simulink model "butterfly_matlab_to_c"  (R2020a)
settings: Solver=FixedStepAuto  StartTime=0.0  StopTime=30  FixedStep=1/120/10  MaxStep=0.01  RelTol=1e-3
undefined symbols (not defined in the file or in its folder): bf
settings Model: SimulationMode=accelerator  Creator=g-oft  LastModifiedBy=g-oft
settings DataIOCC: SaveFormat=StructureWithTime
settings OptimizationCC: OptimizeBlockIOStorage=off  OptimizeDataStoreBuffers=off  BusAssignmentInplaceUpdate=off
settings DebuggingCC: SFUnexpectedBacktrackingDiag=warning  SFNoUnconditionalDefaultTransitionDiag=warning
settings RTWCC: GenerateReport=on  BuildConfiguration=Debug  LaunchReport=on
settings CodeAppCC: ForceParamTrailComments=on  MATLABSourceComments=on  EnableCustomComments=on
settings GRTTargetCC: CombineSignalStateStructs=on  SupportVariableSizeSignals=on  RTWCAPISignals=on  RTWCAPIParams=on  RTWCAPIStates=on  MultiInstanceErrorCode=Warning

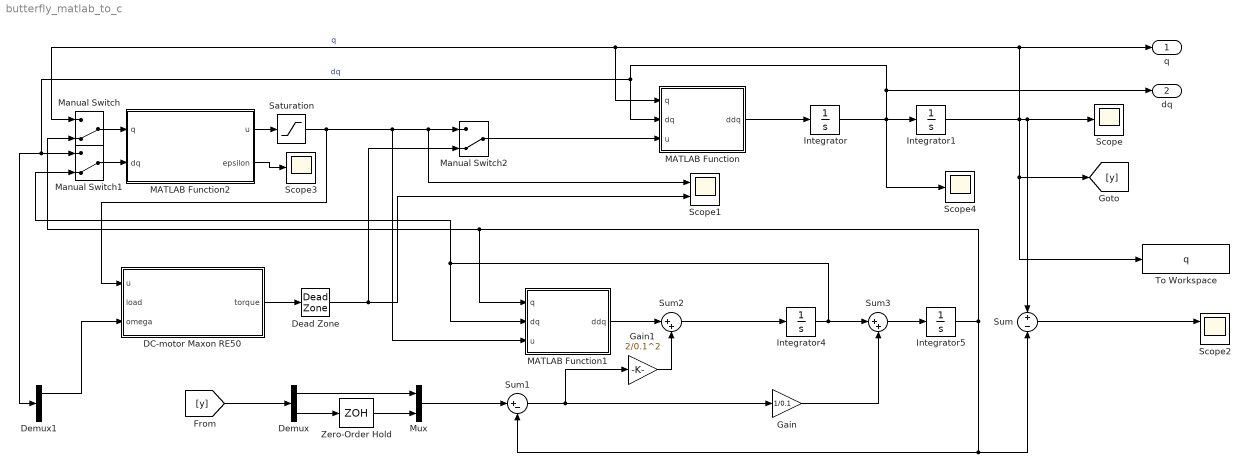
== system butterfly_matlab_to_c ==
  DC-motor Maxon RE50 : Subsystem
  Dead Zone : DeadZone  LowerValue=-5e-3  UpperValue=5e-3  SaturateOnIntegerOverflow=on
  Demux : Demux  Outputs=2
  Demux1 : Demux  Outputs=2
  Gain : Gain  Gain=1/0.1
  Gain1 : Gain  Gain=2/0.1^2
  Integrator : Integrator  InitialCondition=[bf.get_dtheta(0)*bf.function_for_dphi(0);bf.function_for_dphi(0)]
  Integrator1 : Integrator  InitialCondition=[0;0]
  Integrator4 : Integrator  InitialCondition=[0.3;0]
  Integrator5 : Integrator  InitialCondition=[0.1;0]
  MATLAB Function : MATLAB Function  TreatAsAtomicUnit=on
  MATLAB Function1 : MATLAB Function  TreatAsAtomicUnit=on
  MATLAB Function2 : MATLAB Function  TreatAsAtomicUnit=on
  Manual Switch : ManualSwitch  CurrentSetting=0
  Manual Switch1 : ManualSwitch  CurrentSetting=0
  Manual Switch2 : ManualSwitch  CurrentSetting=0
  Mux : Mux  Inputs=2
  Saturation : Saturate  UpperLimit=10  LowerLimit=-10
  Scope : Scope
  Scope1 : Scope  NumInputPorts=2
  Scope2 : Scope  NumInputPorts=2
  Scope3 : Scope
  Scope4 : Scope
  Sum : Sum  Inputs=+-
  Sum1 : Sum  Inputs=|+-
  Sum2 : Sum  Inputs=|++
  Sum3 : Sum  Inputs=|++
  To Workspace : ToWorkspace  VariableName=q  SampleTime=-1
  Zero-Order Hold : ZeroOrderHold  SampleTime=1/120
  q : Outport  SignalName=q
  dq : Outport  Port=2  SignalName=dq
  wires:
  Integrator/1 -> Scope4/1, Integrator1/1, dq/1, Demux1/1, Manual Switch1/1, MATLAB Function/2(dq)  "dq"
  MATLAB Function/1(ddq) -> Integrator/1
  Integrator1/1 -> Sum/1, Scope/1, [y], To Workspace/1, q/1, Manual Switch/1, MATLAB Function/1(q)  "q"
  Integrator4/1 -> MATLAB Function1/2(dq), Manual Switch1/2, Sum3/1
  Sum3/1 -> Integrator5/1
  Integrator5/1 -> Sum/2, Sum1/2, MATLAB Function1/1(q), Manual Switch/2
  Gain1/1 -> Sum2/2
  Gain/1 -> Sum3/2
  MATLAB Function1/1(ddq) -> Sum2/1
  Sum1/1 -> Gain1/1, Gain/1
  Manual Switch1/1 -> MATLAB Function2/2(dq)
  Manual Switch/1 -> MATLAB Function2/1(q)
  Sum2/1 -> Integrator4/1
  Sum/1 -> Scope2/1
  MATLAB Function2/1(u) -> Saturation/1
  DC-motor Maxon RE50/1(torque) -> Dead Zone/1
  Manual Switch2/1 -> MATLAB Function/3(u)
  Saturation/1 -> DC-motor Maxon RE50/1(u), MATLAB Function1/3(u), Scope1/1, Manual Switch2/1
  Demux1/1 -> DC-motor Maxon RE50/3(omega)
  Mux/1 -> Sum1/1
  [y] -> Demux/1
  Zero-Order Hold/1 -> Mux/2
  Demux/2 -> Zero-Order Hold/1
  Demux/1 -> Mux/1
  MATLAB Function2/2(epsilon) -> Scope3/1
  Dead Zone/1 -> Manual Switch2/2, Scope1/2

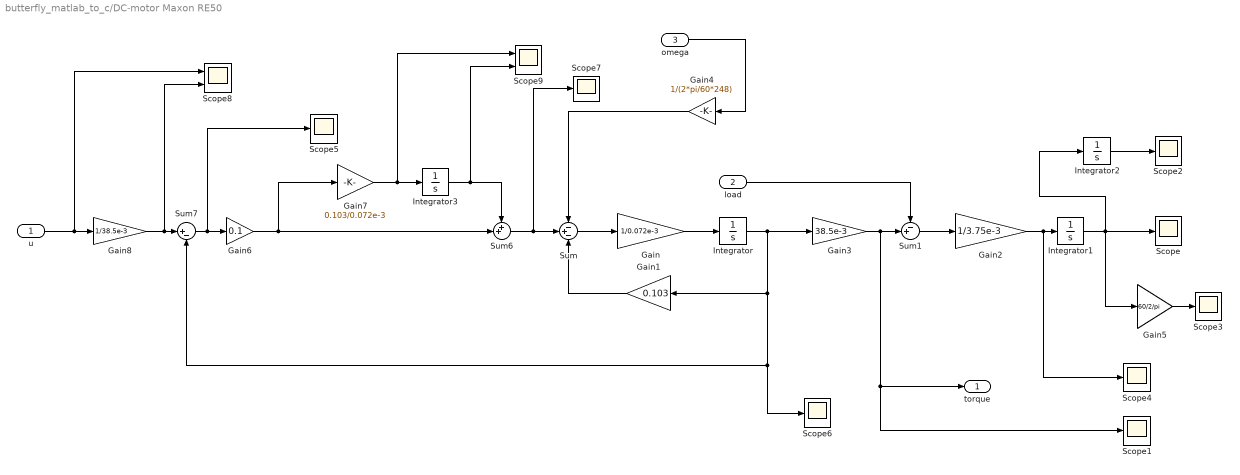
== system butterfly_matlab_to_c/DC-motor Maxon RE50 ==
  u : Inport
  load : Inport  Port=2
  omega : Inport  Port=3
  Gain : Gain  Gain=1/0.072e-3
  Gain1 : Gain  Gain=0.103
  Gain2 : Gain  Gain=1/3.75e-3
  Gain3 : Gain  Gain=38.5e-3
  Gain4 : Gain  Gain=1/(2*pi/60*248)
  Gain5 : Gain  Gain=60/2/pi
  Gain6 : Gain  Gain=0.1
  Gain7 : Gain  Gain=0.103/0.072e-3
  Gain8 : Gain  Gain=1/38.5e-3
  Integrator{,1..3} (4 alike) : Integrator
  Scope{,1..7} (8 alike) : Scope
  Scope8 : Scope  NumInputPorts=2
  Scope9 : Scope  NumInputPorts=2
  Sum : Sum  Inputs=-+-
  Sum1 : Sum  Inputs=-+|
  Sum6 : Sum  Inputs=++|
  Sum7 : Sum  Inputs=|+-
  torque : Outport
  wires:
  Sum/1 -> Gain/1
  Gain/1 -> Integrator/1
  Gain1/1 -> Sum/3
  Sum1/1 -> Gain2/1
  Gain2/1 -> Scope4/1, Integrator1/1
  Gain3/1 -> torque/1, Scope1/1, Sum1/2
  Integrator1/1 -> Gain5/1, Scope/1, Integrator2/1
  Gain4/1 -> Sum/1
  Integrator2/1 -> Scope2/1
  Gain5/1 -> Scope3/1
  Integrator/1 -> Gain1/1, Scope6/1, Sum7/2, Gain3/1
  Integrator3/1 -> Scope9/2, Sum6/1
  Gain6/1 -> Gain7/1, Sum6/2
  Sum7/1 -> Scope5/1, Gain6/1
  Sum6/1 -> Scope7/1, Sum/2
  u/1 -> Scope8/1, Gain8/1
  Gain8/1 -> Scope8/2, Sum7/1
  load/1 -> Sum1/1
  Gain7/1 -> Scope9/1, Integrator3/1
  omega/1 -> Gain4/1

== matlab function butterfly_matlab_to_c/MATLAB Function ==
  settings: updateMethod=DISCRETE
  data: q input; dq input; u input; ddq output
function ddq = calculate_ddq(q,dq,u)
    persistent solutions
    if isempty(solutions)
        solutions = coder.load('solutions_riccati_and_dphi');
    end
    n_varphi = 5000;
    a = 0.1095; %Constant for describing the butterfly frame
    b = 0.0405; %Constant for describing the butterfly frame
    g = 9.81; %Gravity
    J_s = 5.48e-7; %Mass moment of inertia of the ball
    J_f = 1.581e-2; %Mass moment of inertia of the frame, from article.
    m_b = 3.0e-3; %Mass of the ball
    R_b = sqrt(16.55e-3^2-12.5e-3^2); %Radius of the ball
    
    %% Functions relating phi and varphi:
   
    % Temporary using phi = varphi;
    varphi = q(2);
    vartheta = q(1);
    phi = solutions.varphi_to_phi(1,floor(mod(varphi,2*pi)*n_varphi/2/pi)+1);
    

    %% e_phi 
    e_phi = [sin(phi);cos(phi);0];
    d_e_phi = [cos(phi);-sin(phi);0];
    dd_e_phi = [-sin(phi);-cos(phi);0];
    ddd_e_phi = [-cos(phi);sin(phi);0];
    
    %% Delta
    delta = (a-b*cos(2*phi));
    delta_v = delta*e_phi;
    d_delta = b*2*sin(2*phi);
    dd_delta = b*4*cos(2*phi);
    ddd_delta = -b*8*sin(2*phi);
    d_delta_v = d_delta*e_phi+delta*d_e_phi;
    dd_delta_v = dd_delta*e_phi+2*d_delta*d_e_phi+delta*dd_e_phi;
    ddd_delta_v = ddd_delta*e_phi+ 3*dd_delta*d_e_phi + ...
        3*d_delta*dd_e_phi + delta*ddd_e_phi;
    norm_d_delta_v = sqrt(d_delta^2+delta^2);
    
    %% Tau
    tau = d_delta_v/norm_d_delta_v;
    d_tau = dd_delta_v/norm_d_delta_v - d_delta_v*d_delta_v'*dd_delta_v/norm_d_delta_v^3;
    dd_tau = ddd_delta_v/norm_d_delta_v - dd_delta_v*d_delta_v'*dd_delta_v/norm_d_delta_v^3 - ...
        (dd_delta_v*d_delta_v'*dd_delta_v+d_delta_v*(dd_delta_v'*dd_delta_v)+d_delta_v*d_delta_v'*ddd_delta_v)/...
        norm_d_delta_v^3 + d_delta_v*d_delta_v'*dd_delta_v*3*d_delta_v'*dd_delta_v/norm_d_delta_v^5;
    %% Normal vector:
    normal = [0 -1 0;1 0 0;0 0 0]*tau;
    d_normal = [0 -1 0;1 0 0;0 0 0]*d_tau;
    dd_normal = [0 -1 0;1 0 0;0 0 0]*dd_tau;
    

    %% Rho :
    rho = delta_v + R_b*normal;
    d_rho = d_delta_v + R_b*d_normal;
    dd_rho = dd_delta_v + R_b*dd_normal;
    
    %% Need to find varphi = g(phi)
    gamma = delta_v'*[1;0;0]-R_b*tau'*[0;1;0];
    psi = delta_v'*[0;1;0]+R_b*tau'*[1;0;0];
    d_gamma = d_delta_v'*[1;0;0]-R_b*d_tau'*[0;1;0];
    d_psi = d_delta_v'*[0;1;0]+R_b*d_tau'*[1;0;0];
    dd_gamma = dd_delta_v'*[1;0;0]-R_b*dd_tau'*[0;1;0];
    dd_psi = dd_delta_v'*[0;1;0]+R_b*dd_tau'*[1;0;0];
    %func_g = atan2(gamma, psi);
    d_func_g = (d_gamma*psi-d_psi*gamma)/(gamma^2+psi^2);
    dd_func_g = (dd_gamma*psi-dd_psi*gamma)/(psi^2+gamma^2)-(d_gamma*psi-d_psi*gamma)*(2*gamma*d_gamma+2*psi*d_psi)/(gamma^2+psi^2)^2;
    
    %% s
    d_s = norm(d_rho)/d_func_g;
    dd_s = d_rho'*dd_rho/norm(d_rho)/d_func_g^2 - norm(d_rho)*dd_func_g/d_func_g^3;
    
    %% s_f:
    d_sf = norm_d_delta_v/d_func_g;
    dd_sf = d_delta_v'*dd_delta_v/norm_d_delta_v/d_func_g - norm_d_delta_v*dd_func_g/d_func_g^3;
    
    %% Kappa:
    kappa = dd_rho/d_func_g^2/d_s^2;
    
    %% Rotations:
    R = [cos(vartheta) -sin(vartheta) 0;sin(vartheta) cos(vartheta) 0;0 0 1];
    dR = [-sin(vartheta) -cos(vartheta) 0;cos(vartheta) -sin(vartheta) 0;0 0 0];
    
    rhoxtau = cross(rho,tau);
    rhoxkappa = cross(rho,kappa);
    
    m_11 = m_b*(rho'*rho+J_s/m_b+J_f/m_b);
    m_12 = m_b*(d_s*rhoxtau(3)-d_sf*J_s/R_b/m_b);
    m_22 = m_b*(d_s^2+d_sf^2*J_s/R_b^2/m_b);
    M = [m_11 m_12;m_12 m_22];
    
    c_11 = m_b*rho'*tau*d_s*dq(2);
    c_12 = m_b*(rho'*tau*d_s*dq(1)+(dd_s*rhoxtau(3)-dd_sf*J_s/R_b/m_b+d_s^2*rhoxkappa(3))*dq(2));
    c_21 = -m_b*rho'*tau*d_s*dq(1);
    c_22 = m_b*(d_s*dd_s+d_sf*dd_sf*J_s/R_b^2/m_b)*dq(2);
    C = [c_11 c_12;c_21 c_22];
    
    
    G = m_b*[[0 g 0]*dR*rho;[0 g 0]*R*tau*d_s];

    
ddq = M\(-C*[dq(1);dq(2)]-G+[u;0]);

== matlab function butterfly_matlab_to_c/MATLAB Function2 ==
  settings: updateMethod=DISCRETE
  data: q input; u output; dq input; epsilon output
function [u,epsilon] = controller(q,dq)
    
    persistent solutions
    if isempty(solutions)
        solutions = coder.load('solutions_riccati_and_dphi');
    end
    n_varphi = 5000;
    n_riccati_sol = 5000;
    a = 0.1095; %Constant for describing the butterfly frame
    b = 0.0405; %Constant for describing the butterfly frame
    g = 9.81; %Gravity
    J_s = 5.48e-7; %Mass moment of inertia of the ball
    J_f = 1.581e-2; %Mass moment of inertia of the frame, from article.
    m_b = 3.0e-3; %Mass of the ball
    R_b = sqrt(16.55e-3^2-12.5e-3^2); %Radius of the ball
    

    varphi = q(2);

    c1= -6.023940e+01; c2= 9.115470e-03; c3= 1.941337e-03; c4= 1.731620e-03; c5= 7.253528e-04;
    Theta = c1*atan(c2*sin(2*varphi)+c3*sin(4*varphi)+c4*sin(6*varphi)+c5*sin(8*varphi))+varphi;
    d_Theta = c1*(2*c2*cos(2*varphi) + 4*c3*cos(4*varphi) + 6*c4*cos(6*varphi) + 8*c5*cos(8*varphi))/((c2*sin(2*varphi) + c3*sin(4*varphi) + c4*sin(6*varphi) + c5*sin(8*varphi))^2 + 1) + 1;
    dd_Theta = c1*(-4*c2*sin(2*varphi) - 16*c3*sin(4*varphi) - 36*c4*sin(6*varphi) - 64*c5*sin(8*varphi))/((c2*sin(2*varphi) + c3*sin(4*varphi) + c4*sin(6*varphi) + c5*sin(8*varphi))^2 + 1) - 2*c1*(2*c2*cos(2*varphi) + 4*c3*cos(4*varphi) + 6*c4*cos(6*varphi) + 8*c5*cos(8*varphi))^2*(c2*sin(2*varphi) + c3*sin(4*varphi) + c4*sin(6*varphi) + c5*sin(8*varphi))/((c2*sin(2*varphi) + c3*sin(4*varphi) + c4*sin(6*varphi) + c5*sin(8*varphi))^2 + 1)^2;
    
%     c = [0.0024   -0.0383    0.2090   -0.4568    1.3214    0.0055];
%     x = varphi;
%     phi = varphi;%c*[x^5;x^4;x^3;x^2;x;1];
    phi = solutions.varphi_to_phi(1,floor(mod(varphi,2*pi)*n_varphi/2/pi)+1);
    vartheta = Theta;
    d_vartheta = d_Theta*dq(2);
    
    %% e_phi 
    e_phi = [sin(phi);cos(phi);0];
    d_e_phi = [cos(phi);-sin(phi);0];
    dd_e_phi = [-sin(phi);-cos(phi);0];
    ddd_e_phi = [-cos(phi);sin(phi);0];
    
    %% Delta
    delta = (a-b*cos(2*phi));
    delta_v = delta*e_phi;
    d_delta = b*2*sin(2*phi);
    dd_delta = b*4*cos(2*phi);
    ddd_delta = -b*8*sin(2*phi);
    d_delta_v = d_delta*e_phi+delta*d_e_phi;
    dd_delta_v = dd_delta*e_phi+2*d_delta*d_e_phi+delta*dd_e_phi;
    ddd_delta_v = ddd_delta*e_phi+ 3*dd_delta*d_e_phi + ...
        3*d_delta*dd_e_phi + delta*ddd_e_phi;
    norm_d_delta_v = sqrt(d_delta^2+delta^2);
    
    %% Tau
    tau = d_delta_v/norm_d_delta_v;
    d_tau = dd_delta_v/norm_d_delta_v - d_delta_v*d_delta_v'*dd_delta_v/norm_d_delta_v^3;
    dd_tau = ddd_delta_v/norm_d_delta_v - dd_delta_v*d_delta_v'*dd_delta_v/norm_d_delta_v^3 - ...
        (dd_delta_v*d_delta_v'*dd_delta_v+d_delta_v*(dd_delta_v'*dd_delta_v)+d_delta_v*d_delta_v'*ddd_delta_v)/...
        norm_d_delta_v^3 + d_delta_v*d_delta_v'*dd_delta_v*3*d_delta_v'*dd_delta_v/norm_d_delta_v^5;
    %% Normal vector:
    normal = [0 -1 0;1 0 0;0 0 0]*tau;
    d_normal = [0 -1 0;1 0 0;0 0 0]*d_tau;
    dd_normal = [0 -1 0;1 0 0;0 0 0]*dd_tau;
    

    %% Rho :
    rho = delta_v + R_b*normal;
    d_rho = d_delta_v + R_b*d_normal;
    dd_rho = dd_delta_v + R_b*dd_normal;
    
    %% Need to find varphi = g(phi)
    gamma = delta_v'*[1;0;0]-R_b*tau'*[0;1;0];
    psi = delta_v'*[0;1;0]+R_b*tau'*[1;0;0];
    d_gamma = d_delta_v'*[1;0;0]-R_b*d_tau'*[0;1;0];
    d_psi = d_delta_v'*[0;1;0]+R_b*d_tau'*[1;0;0];
    dd_gamma = dd_delta_v'*[1;0;0]-R_b*dd_tau'*[0;1;0];
    dd_psi = dd_delta_v'*[0;1;0]+R_b*dd_tau'*[1;0;0];
    %func_g = atan2(gamma, psi);
    d_func_g = (d_gamma*psi-d_psi*gamma)/(gamma^2+psi^2);
    dd_func_g = (dd_gamma*psi-dd_psi*gamma)/(psi^2+gamma^2)-(d_gamma*psi-d_psi*gamma)*(2*gamma*d_gamma+2*psi*d_psi)/(gamma^2+psi^2)^2;
    
    %% s
    d_s = norm(d_rho)/d_func_g;
    dd_s = d_rho'*dd_rho/norm(d_rho)/d_func_g^2 - norm(d_rho)*dd_func_g/d_func_g^3;
    
    %% s_f:
    d_sf = norm_d_delta_v/d_func_g;
    dd_sf = d_delta_v'*dd_delta_v/norm_d_delta_v/d_func_g - norm_d_delta_v*dd_func_g/d_func_g^3;
    
    %% Kappa:
    kappa = dd_rho/d_func_g^2/d_s^2;
    
    %% Rotations:
    R = [cos(vartheta) -sin(vartheta) 0;sin(vartheta) cos(vartheta) 0;0 0 1];
    dR = [-sin(vartheta) -cos(vartheta) 0;cos(vartheta) -sin(vartheta) 0;0 0 0];
    
    rhoxtau = cross(rho,tau);
    rhoxkappa = cross(rho,kappa);
    
    m_11 = m_b*(rho'*rho+J_s/m_b+J_f/m_b);
    m_12 = m_b*(d_s*rhoxtau(3)-d_sf*J_s/R_b/m_b);
    m_22 = m_b*(d_s^2+d_sf^2*J_s/R_b^2/m_b);
    M = [m_11 m_12;m_12 m_22];
    
    c_11 = m_b*rho'*tau*d_s*dq(2);
    c_12 = m_b*(rho'*tau*d_s*d_vartheta+(dd_s*rhoxtau(3)-dd_sf*J_s/R_b/m_b+d_s^2*rhoxkappa(3))*dq(2));
    c_21 = -m_b*rho'*tau*d_s*d_vartheta;
    c_22 = m_b*(d_s*dd_s+d_sf*dd_sf*J_s/R_b^2/m_b)*dq(2);
    C = [c_11 c_12;c_21 c_22];
    
    G = m_b*[[0 g 0]*dR*rho;[0 g 0]*R*tau*d_s];
    
    d_phi_star = solutions.d_phi_star(1,floor(mod(q(2),pi)*n_riccati_sol/pi)+1);
    riccati_sol = solutions.riccati_sol(:,:,floor(mod(q(2),pi)*n_riccati_sol/pi)+1);
    
    alpha = m_b*((d_s*rhoxtau(3)-d_sf*J_s/R_b/m_b)*d_Theta+d_s^2+d_sf^2*J_s/R_b/m_b/R_b);
%     beta = m_b*((d_s*rhoxtau(3)-d_sf*J_s/R_b/m_b)*dd_Theta-rho'*tau*d_s*d_Theta^2 ...
%         + d_s*dd_s + d_sf*dd_sf*J_s/R_b/m_b/R_b);
%     gamma = m_b*[0 g 0]*R*tau*d_s;

    g_w = -m_b*(d_s*rhoxtau(3)-d_sf*J_s/m_b/R_b);
%     g_y_dot = m_b*d_s*tau'*rho*(2*d_Theta*d_varphi);
%     g_y = -get_ds(varphi)*m_b*g*[cos(get_theta(varphi)) -sin(get_theta(varphi)) 0]*get_tau(varphi);
%     
    B = [0;1;g_w/alpha];
    Gamma = 1;
    epsilon = [q(1)-Theta;dq(1)-d_Theta*dq(2);dq(2)-d_phi_star];
    
    w = -(1/Gamma)*B'*riccati_sol*epsilon;
    
    k = [1 0]*M*[d_Theta;1]/([d_Theta 1]*M*[0;1]);
    
u = k*([k^-1 -1]*M*[w+dd_Theta*dq(2)^2;0]+[k^-1 -1]*C*[d_Theta*dq(2)+epsilon(2);dq(2)]+[k^-1 -1]*G);

== matlab function butterfly_matlab_to_c/MATLAB Function1 ==
  settings: updateMethod=DISCRETE
  data: q input; dq input; u input; ddq output
function ddq = calculate_ddq(q,dq,u)
    persistent solutions
    if isempty(solutions)
        solutions = coder.load('solutions_riccati_and_dphi');
    end
    n_varphi = 5000;
    a = 0.1095; %Constant for describing the butterfly frame
    b = 0.0405; %Constant for describing the butterfly frame
    g = 9.81; %Gravity
    J_s = 5.48e-7; %Mass moment of inertia of the ball
    J_f = 1.581e-2; %Mass moment of inertia of the frame, from article.
    m_b = 3.0e-3; %Mass of the ball
    R_b = sqrt(16.55e-3^2-12.5e-3^2); %Radius of the ball
    
    %% Functions relating phi and varphi:
   
    % Temporary using phi = varphi;
    varphi = q(2);
    vartheta = q(1);
    phi = solutions.varphi_to_phi(1,floor(mod(varphi,2*pi)*n_varphi/2/pi)+1);
    

    %% e_phi 
    e_phi = [sin(phi);cos(phi);0];
    d_e_phi = [cos(phi);-sin(phi);0];
    dd_e_phi = [-sin(phi);-cos(phi);0];
    ddd_e_phi = [-cos(phi);sin(phi);0];
    
    %% Delta
    delta = (a-b*cos(2*phi));
    delta_v = delta*e_phi;
    d_delta = b*2*sin(2*phi);
    dd_delta = b*4*cos(2*phi);
    ddd_delta = -b*8*sin(2*phi);
    d_delta_v = d_delta*e_phi+delta*d_e_phi;
    dd_delta_v = dd_delta*e_phi+2*d_delta*d_e_phi+delta*dd_e_phi;
    ddd_delta_v = ddd_delta*e_phi+ 3*dd_delta*d_e_phi + ...
        3*d_delta*dd_e_phi + delta*ddd_e_phi;
    norm_d_delta_v = sqrt(d_delta^2+delta^2);
    
    %% Tau
    tau = d_delta_v/norm_d_delta_v;
    d_tau = dd_delta_v/norm_d_delta_v - d_delta_v*d_delta_v'*dd_delta_v/norm_d_delta_v^3;
    dd_tau = ddd_delta_v/norm_d_delta_v - dd_delta_v*d_delta_v'*dd_delta_v/norm_d_delta_v^3 - ...
        (dd_delta_v*d_delta_v'*dd_delta_v+d_delta_v*(dd_delta_v'*dd_delta_v)+d_delta_v*d_delta_v'*ddd_delta_v)/...
        norm_d_delta_v^3 + d_delta_v*d_delta_v'*dd_delta_v*3*d_delta_v'*dd_delta_v/norm_d_delta_v^5;
    %% Normal vector:
    normal = [0 -1 0;1 0 0;0 0 0]*tau;
    d_normal = [0 -1 0;1 0 0;0 0 0]*d_tau;
    dd_normal = [0 -1 0;1 0 0;0 0 0]*dd_tau;
    

    %% Rho :
    rho = delta_v + R_b*normal;
    d_rho = d_delta_v + R_b*d_normal;
    dd_rho = dd_delta_v + R_b*dd_normal;
    
    %% Need to find varphi = g(phi)
    gamma = delta_v'*[1;0;0]-R_b*tau'*[0;1;0];
    psi = delta_v'*[0;1;0]+R_b*tau'*[1;0;0];
    d_gamma = d_delta_v'*[1;0;0]-R_b*d_tau'*[0;1;0];
    d_psi = d_delta_v'*[0;1;0]+R_b*d_tau'*[1;0;0];
    dd_gamma = dd_delta_v'*[1;0;0]-R_b*dd_tau'*[0;1;0];
    dd_psi = dd_delta_v'*[0;1;0]+R_b*dd_tau'*[1;0;0];
    %func_g = atan2(gamma, psi);
    d_func_g = (d_gamma*psi-d_psi*gamma)/(gamma^2+psi^2);
    dd_func_g = (dd_gamma*psi-dd_psi*gamma)/(psi^2+gamma^2)-(d_gamma*psi-d_psi*gamma)*(2*gamma*d_gamma+2*psi*d_psi)/(gamma^2+psi^2)^2;
    
    %% s
    d_s = norm(d_rho)/d_func_g;
    dd_s = d_rho'*dd_rho/norm(d_rho)/d_func_g^2 - norm(d_rho)*dd_func_g/d_func_g^3;
    
    %% s_f:
    d_sf = norm_d_delta_v/d_func_g;
    dd_sf = d_delta_v'*dd_delta_v/norm_d_delta_v/d_func_g - norm_d_delta_v*dd_func_g/d_func_g^3;
    
    %% Kappa:
    kappa = dd_rho/d_func_g^2/d_s^2;
    
    %% Rotations:
    R = [cos(vartheta) -sin(vartheta) 0;sin(vartheta) cos(vartheta) 0;0 0 1];
    dR = [-sin(vartheta) -cos(vartheta) 0;cos(vartheta) -sin(vartheta) 0;0 0 0];
    
    rhoxtau = cross(rho,tau);
    rhoxkappa = cross(rho,kappa);
    
    m_11 = m_b*(rho'*rho+J_s/m_b+J_f/m_b);
    m_12 = m_b*(d_s*rhoxtau(3)-d_sf*J_s/R_b/m_b);
    m_22 = m_b*(d_s^2+d_sf^2*J_s/R_b^2/m_b);
    M = [m_11 m_12;m_12 m_22];
    
    c_11 = m_b*rho'*tau*d_s*dq(2);
    c_12 = m_b*(rho'*tau*d_s*dq(1)+(dd_s*rhoxtau(3)-dd_sf*J_s/R_b/m_b+d_s^2*rhoxkappa(3))*dq(2));
    c_21 = -m_b*rho'*tau*d_s*dq(1);
    c_22 = m_b*(d_s*dd_s+d_sf*dd_sf*J_s/R_b^2/m_b)*dq(2);
    C = [c_11 c_12;c_21 c_22];
    
    
    G = m_b*[[0 g 0]*dR*rho;[0 g 0]*R*tau*d_s];

    
ddq = M\(-C*[dq(1);dq(2)]-G+[u;0]);
